simulink model "SimulinkVehicle"  (R2024a)
settings: Solver=FixedStepAuto  StartTime=0  StopTime=1000  FixedStep=simStepSize  RelTol=1e-3
PreLoadFcn:
  | % To support Reader and Writer blocks, some bus objects must be loaded
  | load(fullfile(matlabroot,'toolbox','driving','drivingdata','rrScenarioSimTypes.mat'));
undefined symbols (not defined in the file or in its folder): gainArg, simStepSize
libraries: roadrunnerscenario x1
settings Model: Creator=The MathWorks, Inc.  LastModifiedBy=fukuchi
settings SolverCC: MaxZcPerStep=1
settings DataIOCC: SaveOutput=off  DSMLogging=off  SaveTime=off  ReturnWorkspaceOutputs=off
settings ModelReferenceCC: EnableRefExpFcnMdlSchedulingChecks=on
settings RTWCC: GPUComputeCapability=3.5  DLArmComputeVersion=19.05

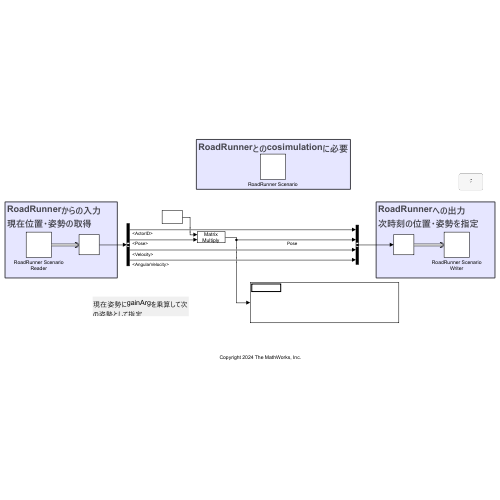
[thumbnail: Simulink's stored preview of the top-level diagram]
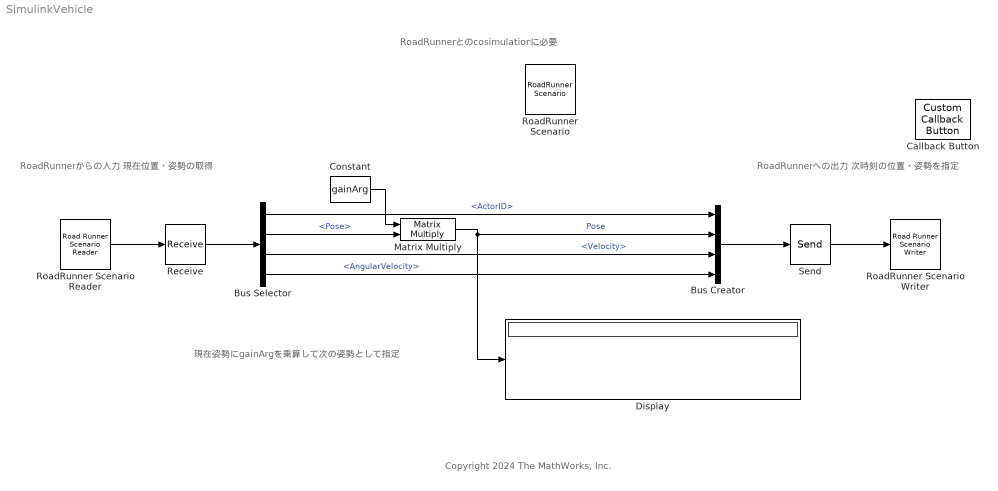
== system SimulinkVehicle ==
  note: 現在姿勢にgainArgを乗算して次の姿勢として指定
  note: RoadRunnerとのcosimulationに必要
  note: Copyright 2024 The MathWorks, Inc.
  note: RoadRunnerからの入力
      | 現在位置・姿勢の取得
  note: RoadRunnerへの出力
      | 次時刻の位置・姿勢を指定
  Bus Creator : BusCreator  Inputs=4  OutDataTypeStr=Bus: BusActorRuntime  NonVirtualBus=on
  Bus Selector : BusSelector  OutputSignals=ActorID,Pose,Velocity,AngularVelocity
  Callback Button : CustomCallbackButton  Configuration="{\"components\":[{\"name\":\"BackgroundImageComponent\",\"settings\":{\"image\":{\"size\":[0,0],\"src\":\"default\",\"srcOrientation\":\"Right\"},\"position\":[0,0,1,1]}},{\"name\":\"ButtonStateComponent\",\"settings\":{\"buttonType\":\"momentary\",\"clickFcn\":\"helpview('driving','SimulateRoadRunnerwithSimulink')\",\"onValue\":1,\"position\":[0,0,1,1],\"pressDelay\":\"500\",\"pressFcn\":\"\",\"repeatInterval\":\"0\",\"states\":[{\"horizontalAlignment\":\"center\",\"image\":{\"position\":[0,0,1,1],\"src\":\"default\",\"srcOrientation\":\"Right\"},\"label\":{\"color\":[0.01176470588,0.01176470588,0.01176470588,1],\"icon\":{\"size\":[0,0],\"src\":\"default\",\"srcOrientation\":\"Right\"},\"iconPlacement\":\"left\",\"text\":{\"content\":\"?\"}},\"labelOffset\":[0,0],\"verticalAlignment\":\"middle\"},{\"horizontalAlignment\":\"center\",\"image\":{\"position\":[0,0,1,1],\"src\":\"default\",\"srcOrientation\":\"Right\"},\"label\":{\"color\":[0.01176470588,0.01176470588,0.01176470588,1],\"icon\":{\"size\":[0,0],\"src\":\"default\",\"srcOrientation\":\"Right\"},\"iconPlacement\":\"left\",\"text\":{\"content\":\"?\"}},\"labelOffset\":[0,0],\"verticalAlignment\":\"middle\"},{\"horizontalAlignment\":\"center\",\"image\":{\"position\":[0,0,1,1],\"src\":\"default\",\"srcOrientation\":\"Right\"},\"label\":{\"color\":[0.01176470588,0.01176470588,0.01176470588,1],\"icon\":{\"size\":[0,0],\"src\":\"default\",\"srcOrientation\":\"Right\"},\"iconPlacement\":\"left\",\"text\":{\"content\":\"?\"}},\"labelOffset\":[0,0],\"verticalAlignment\":\"middle\"},{\"horizontalAlignment\":\"center\",\"image\":{\"position\":[0,0,1,1],\"src\":\"default\",\"srcOrientation\":\"Right\"},\"label\":{\"color\":[0.01176470588,0.01176470588,0.01176470588,1],\"icon\":{\"size\":[0,0],\"src\":\"default\",\"srcOrientation\":\"Right\"},\"iconPlacement\":\"left\",\"text\":{\"content\":\"?\"}},\"labelOffset\":[0,0],\"verticalAlignment\":\"middle\"}]}},{\"name\":\"ForegroundImageComponent\",\"settings\":{\"image\":{\"size\":[0,0],\"src\":\"default\",\"srcOrientation\":\"Right\"},\"isForeground\":1,\"position\":[0,0,1,1]}}],\"settings\":{\"BindingType\":\"standalone\",\"backgroundColor\":[244,244,244,1],\"backgroundOffset\":0.2,\"backgroundOpacity\":1,\"fixedAspectRatio\":\"off\",\"foregroundColor\":[0.01176470588,0.01176470588,0.01176470588,1],\"migratedFromLegacy\":true,\"useBackgroundColor\":true,\"variant\":\"callback\",\"version\":\"R2023a\"},\"type\":\"Button\"}"  CustomBackgroundColor="{\"color\":[0.9568627451,0.9568627451,0.9568627451],\"show\":true}"
  Constant : Constant  Value=gainArg  VectorParams1D=off
  Display : Display
  Matrix Multiply : Product  Multiplication=Matrix(*)
  Receive : Receive  InputPortMessageModes=m  UseInternalQueue=off  QueueOverwriting=on  QueueLength=1  QueueType=LIFO
  RoadRunner Scenario : roadrunnerscenario/RoadRunner Scenario  UserDefinedActions={}  UserDefinedEvents={}
  RoadRunner Scenario Reader : RoadRunnerScenarioReader  OutputPortMessageModes=m  TopicType=Actor Pose  VehicleType=Vehicle Specifications  SampleTime=simStepSize
  RoadRunner Scenario Writer : RoadRunnerScenarioWriter  InputPortMessageModes=m  TopicType=Actor Pose  VehicleType=Vehicle Pose
  Send : Send  OutputPortMessageModes=m
  wires:
  RoadRunner Scenario Reader/1 -> Receive/1
  Receive/1 -> Bus Selector/1
  Bus Creator/1 -> Send/1
  Bus Selector/1 -> Bus Creator/1  "<ActorID>"
  Bus Selector/4 -> Bus Creator/4  "<AngularVelocity>"
  Bus Selector/2 -> Matrix Multiply/2  "<Pose>"
  Constant/1 -> Matrix Multiply/1
  Matrix Multiply/1 -> Bus Creator/2, Display/1  "Pose"
  Send/1 -> RoadRunner Scenario Writer/1
  Bus Selector/3 -> Bus Creator/3  "<Velocity>"
